simulink model "CCCV"  (R2019a)
settings: Solver=FixedStepAuto  StartTime=0.0  StopTime=3600  FixedStep=0.1  RelTol=1e-3
undefined symbols (not defined in the file or in its folder): x0_nom
settings Model: Creator=ztakeo  LastModifiedBy=ztakeo

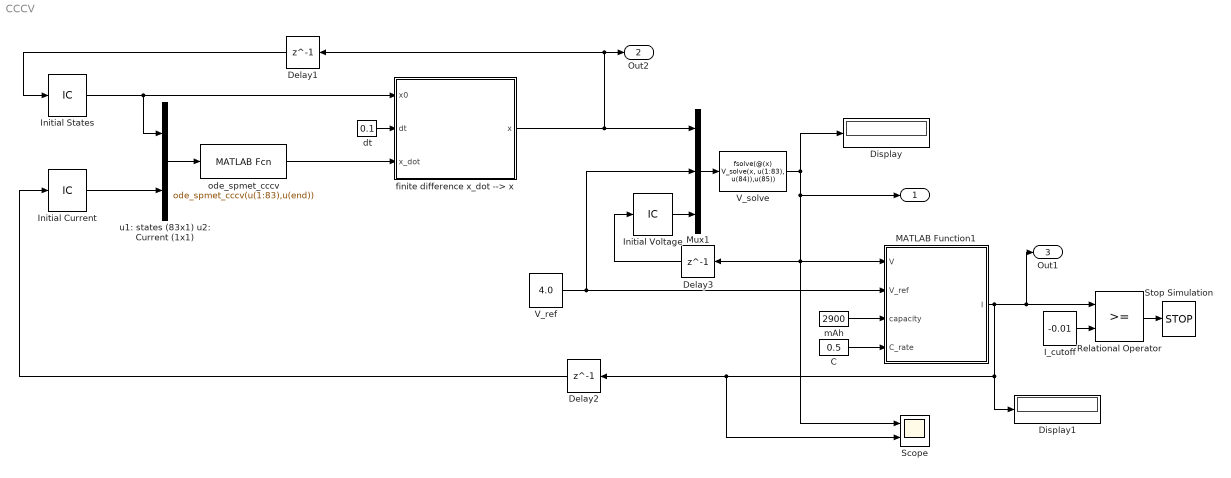
== system CCCV ==
  C : Constant  Value=0.5
  Delay1 : Delay  DelayLength=1  InitialCondition=0
  Delay2 : Delay  DelayLength=1  InitialCondition=0
  Delay3 : Delay  DelayLength=1  InitialCondition=0
  Display : Display
  Display1 : Display
  I_cutoff : Constant  Value=-0.01
  Initial Current : InitialCondition  Value=0
  "Initial States " : InitialCondition  Value=x0_nom
  "Initial Voltage " : InitialCondition  Value=2.8
  MATLAB Function1 : MATLAB Function  TreatAsAtomicUnit=on
  Mux1 : Mux  Inputs=3
  Relational Operator : RelationalOperator  OutDataTypeStr=boolean  RndMeth=Simplest
  Scope : Scope  NumInputPorts=2
  Stop Simulation : Stop
  "V_ref " : Constant  Value=4.0
  V_solve : MATLABFcn  MATLABFcn=fsolve(@(x) V_solve(x, u(1:83), u(84)),u(85))  OutputDimensions=1
  dt : Constant  Value=0.1
  finite difference x_dot --> x : MATLAB Function  TreatAsAtomicUnit=on
  mAh : Constant  Value=2900
  ode_spmet_cccv : MATLABFcn  MATLABFcn=ode_spmet_cccv(u(1:83),u(end))  OutputDimensions=83  OutputSignalType=real
  u1: states (83x1) u2: Current (1x1) : Mux  Inputs=2
  " " : Outport  SignalName=V
  Out2 : Outport  Port=2  SignalName=x
  Out1 : Outport  Port=3  SignalName=Current
  wires:
  Mux1/1 -> V_solve/1
  "V_ref "/1 -> MATLAB Function1/2(V_ref), Mux1/2
  dt/1 -> finite difference x_dot --> x/2(dt)
  u1: states (83x1) u2: Current (1x1)/1 -> ode_spmet_cccv/1
  "Initial States "/1 -> u1: states (83x1) u2: Current (1x1)/1, finite difference x_dot --> x/1(x0)
  Relational Operator/1 -> Stop Simulation/1
  I_cutoff/1 -> Relational Operator/2
  "Initial Voltage "/1 -> Mux1/3
  Initial Current/1 -> u1: states (83x1) u2: Current (1x1)/2
  ode_spmet_cccv/1 -> finite difference x_dot --> x/3(x_dot)
  finite difference x_dot --> x/1(x) -> Delay1/1, Out2/1, Mux1/1
  V_solve/1 -> Scope/1, Delay3/1, MATLAB Function1/1(V), " "/1, Display/1
  MATLAB Function1/1(I) -> Scope/2, Delay2/1, Display1/1, Out1/1, Relational Operator/1
  Delay2/1 -> Initial Current/1
  Delay1/1 -> "Initial States "/1
  Delay3/1 -> "Initial Voltage "/1
  mAh/1 -> MATLAB Function1/3(capacity)
  C/1 -> MATLAB Function1/4(C_rate)

== matlab function CCCV/MATLAB Function1 ==
  data: V input; V_ref input; I output; capacity input; C_rate input
%% PI Controller function
function I = fcn(V,V_ref,capacity,C_rate)
    I_chrgmax = -capacity*C_rate/1000; %A

    Kp = 10;
    
    % Compute control law current, but regulate if above max charge rate
    I_ctrl = Kp*(V-V_ref);
    
    if I_ctrl < I_chrgmax % charging current is negative, so higher charging rate is a more negative value
        scale_Kp = I_chrgmax/I_ctrl; % bound the max current; here use max instead of min because charge current is (-)
        % recompute Kp if         
        I = scale_Kp*Kp*(V-V_ref);
    else % case where charging current from controller doesn't exceed max rate
        I = I_ctrl;
    end

end

== matlab function CCCV/finite difference x_dot --> x ==
  data: x0 input; x output; dt input; x_dot input
%% Simple function for stepping forward based on finite difference scheme
function x = fcn(x0,dt,x_dot)
    x = x0 + dt*x_dot;
end
